simulink model "fullVehicleModel_17b"  (R2017b)
settings: Solver=VariableStepAuto  StartTime=0.0  StopTime=10.0  RelTol=1e-3
undefined symbols (not defined in the file): ambient_temp, bat, bat_r1, Batt, batt_initCharge, Batt_sensorLag_s, bvatt_AhRating, DiscIntNeverNeededParam, electronics_power, env, module_broad_area, module_small_area, module_top_area, mot, no_module, shifterPos, Ts, Ts_elec
libraries: Soft_ECUs x90, fl_lib x67, nesl_utility x29, Battery_lib x28, Gen_lib x13, simulink x10, aerolibconvert2 x7, SoftCAN_Interface x6, autolibshared x2, Additional_blocks_lib x1, elec_lib x1
(part 2 of 4)

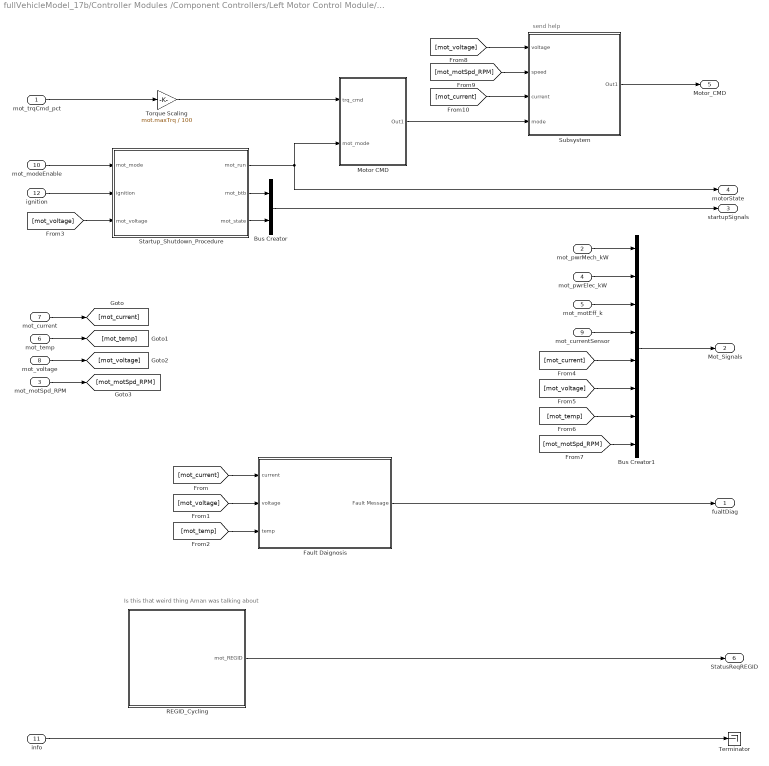
== system fullVehicleModel_17b/Controller Modules /Component Controllers/Left Motor Control Module/Controller ==
  note: send help
  note: Is this that weird thing Aman was talking about
  mot_trqCmd_pct : Inport
  mot_pwrMech_kW : Inport  Port=2
  mot_motSpd_RPM : Inport  Port=3
  mot_pwrElec_kW : Inport  Port=4
  mot_motEff_k : Inport  Port=5
  mot_temp : Inport  Port=6
  mot_current : Inport  Port=7
  mot_voltage : Inport  Port=8
  mot_currentSensor : Inport  Port=9
  mot_modeEnable : Inport  Port=10
  info : Inport  Port=11
  ignition : Inport  Port=12
  Bus Creator : BusCreator  Inputs=2
  Bus Creator1 : BusCreator  Inputs=8
  Fault Daignosis : Subsystem  AncestorBlock=Soft_ECUs/softECU_Motor/Fault Daignosis
  Motor CMD : Subsystem
  REGID_Cycling : Stateflow chart  TreatAsAtomicUnit=on
  Startup_Shutdown_Procedure : Stateflow chart  AncestorBlock=Soft_ECUs/softECU_Motor/Startup_Shutdown_Procedure  TreatAsAtomicUnit=on
  Subsystem : Subsystem
  Terminator : Terminator
  Torque Scaling : Gain  Gain=mot.maxTrq / 100
  fualtDiag : Outport
  Mot_Signals : Outport  Port=2
  startupSignals : Outport  Port=3
  motorState : Outport  Port=4
  Motor_CMD : Outport  Port=5
  StatusReqREGID : Outport  Port=6
  wires:
  mot_modeEnable/1 -> Startup_Shutdown_Procedure/1(mot_mode)
  ignition/1 -> Startup_Shutdown_Procedure/2(ignition)
  mot_trqCmd_pct/1 -> Torque Scaling/1
  Torque Scaling/1 -> Motor CMD/1(trq_cmd)
  Motor CMD/1(Out1) -> Subsystem/4(mode)
  Startup_Shutdown_Procedure/1(mot_run) -> motorState/1, Motor CMD/2(mot_mode)
  Fault Daignosis/1(Fault Message) -> fualtDiag/1
  Subsystem/1(Out1) -> Motor_CMD/1
  Startup_Shutdown_Procedure/2(mot_btb) -> Bus Creator/1
  Startup_Shutdown_Procedure/3(mot_state) -> Bus Creator/2
  Bus Creator/1 -> startupSignals/1
  REGID_Cycling/1(mot_REGID) -> StatusReqREGID/1
  mot_current/1 -> [mot_current]
  mot_voltage/1 -> [mot_voltage]
  mot_temp/1 -> [mot_temp]
  mot_motSpd_RPM/1 -> [mot_motSpd_RPM]
  mot_pwrMech_kW/1 -> Bus Creator1/1
  [mot_current] -> Fault Daignosis/1(current)
  mot_currentSensor/1 -> Bus Creator1/4
  mot_pwrElec_kW/1 -> Bus Creator1/2
  mot_motEff_k/1 -> Bus Creator1/3
  [mot_voltage] -> Fault Daignosis/2(voltage)
  [mot_temp] -> Fault Daignosis/3(temp)
  [mot_voltage] -> Startup_Shutdown_Procedure/3(mot_voltage)
  Bus Creator1/1 -> Mot_Signals/1
  [mot_current] -> Bus Creator1/5
  [mot_voltage] -> Bus Creator1/6
  [mot_temp] -> Bus Creator1/7
  [mot_motSpd_RPM] -> Bus Creator1/8
  [mot_voltage] -> Subsystem/1(voltage)
  [mot_motSpd_RPM] -> Subsystem/2(speed)
  [mot_current] -> Subsystem/3(current)
  info/1 -> Terminator/1

== system fullVehicleModel_17b/Controller Modules /Component Controllers/Left Motor Control Module/Controller Inputs ==
  note: 1) Add Subsystem or Model blocks as valid variant choices.
      | 2) You cannot connect blocks at this level. At simulation, connectivity is automatically
      | determined, based on the active variant and port name matching.
  HSC Inputs : Inport
  Motor Signals : Inport  Port=2
  Ignition : Inport  Port=3
  SiL Inputs : Subsystem  VariantControl=Variant
  mot_trqCmd_pct : Outport
  mot_pwrMech_kW : Outport  Port=2
  mot_motSpd_RPM : Outport  Port=3
  mot_pwrElec_kW : Outport  Port=4
  mot_motEff_k : Outport  Port=5
  mot_temp : Outport  Port=6
  mot_current : Outport  Port=7
  mot_voltage : Outport  Port=8
  mot_currentSensor : Outport  Port=9
  mot_modeEnable : Outport  Port=10
  Info : Outport  Port=11
  Ignition1 : Outport  Port=12

== system fullVehicleModel_17b/Controller Modules /Component Controllers/Left Motor Control Module/Controller Outputs ==
  note: 1) Add Subsystem or Model blocks as valid variant choices.
      | 2) You cannot connect blocks at this level. At simulation, connectivity is automatically
      | determined, based on the active variant and port name matching.
  FaultDiagnos : Inport
  MotorSignals : Inport  Port=2
  StartupSignals : Inport  Port=3
  MotorState : Inport  Port=4
  MotorCMD : Inport  Port=5
  StatusRequest : Inport  Port=6
  SiL Controller Outputs : Subsystem  VariantControl=Variant
  MotorToHSC : Outport
  MotorTrqCMD : Outport  Port=2

== system fullVehicleModel_17b/Controller Modules /Component Controllers/Right Motor Control Module/Controller Inputs ==
  note: 1) Add Subsystem or Model blocks as valid variant choices.
      | 2) You cannot connect blocks at this level. At simulation, connectivity is automatically
      | determined, based on the active variant and port name matching.
  In1 : Inport
  In2 : Inport  Port=2
  In3 : Inport  Port=3
  SiL Inputs : Subsystem  VariantControl=Variant
  Out1 : Outport
  Out2 : Outport  Port=2
  Out3 : Outport  Port=3
  Out4 : Outport  Port=4
  Out5 : Outport  Port=5
  Out6 : Outport  Port=6
  Out7 : Outport  Port=7
  Out8 : Outport  Port=8
  Out9 : Outport  Port=9
  Out10 : Outport  Port=10
  Out11 : Outport  Port=11
  Out12 : Outport  Port=12

== system fullVehicleModel_17b/Controller Modules /Component Controllers/Right Motor Control Module/Controller Outputs ==
  note: 1) Add Subsystem or Model blocks as valid variant choices.
      | 2) You cannot connect blocks at this level. At simulation, connectivity is automatically
      | determined, based on the active variant and port name matching.
  FaultDiagnos : Inport
  MotorSignals : Inport  Port=2
  StartupSignals : Inport  Port=3
  MotorState : Inport  Port=4
  MotorCMD : Inport  Port=5
  StatusRequest : Inport  Port=6
  SiL Controller Outputs : Subsystem  VariantControl=Variant
  MotorToHSC : Outport
  MotorTrqCMD : Outport  Port=2

== system fullVehicleModel_17b/Controller Modules /Component Controllers/Right Motor Control Module/Subsystem ==
  In1 : Inport
  In2 : Inport  Port=2
  In3 : Inport  Port=3
  In4 : Inport  Port=4
  In5 : Inport  Port=5
  In6 : Inport  Port=6
  In7 : Inport  Port=7
  In8 : Inport  Port=8
  In9 : Inport  Port=9
  In10 : Inport  Port=10
  In11 : Inport  Port=11
  In12 : Inport  Port=12
  Out1 : Outport
  Out2 : Outport  Port=2
  Out3 : Outport  Port=3
  Out4 : Outport  Port=4
  Out5 : Outport  Port=5
  Out6 : Outport  Port=6

== system fullVehicleModel_17b/Longitudinal Driver/Driver Model/Driver Model/Classic Driver ==
  CmdVel : Inport
  "Grade " : Inport  Port=2
  VelFdbk : Inport  Port=3
  Longitudinal Driver : autolibshared/Longitudinal Driver  vnom=100  Kp=15  Ki=1  Kaw=.1  Kff=.05  Kg=.01  tauerr=.03
      settings: SourceProductName=Powertrain Blockset  SourceProductBaseCode=PW
  Terminator : Terminator
  AccelCmd : Outport
  BrkCmd : Outport  Port=2
  wires:
  Longitudinal Driver/3 -> BrkCmd/1
  CmdVel/1 -> Longitudinal Driver/1
  VelFdbk/1 -> Longitudinal Driver/2
  "Grade "/1 -> Longitudinal Driver/3
  Longitudinal Driver/2 -> AccelCmd/1
  Longitudinal Driver/1 -> Terminator/1

== system fullVehicleModel_17b/Longitudinal Driver/Driver Model/Driver Model/Thermostatic Driver ==
  CmdVel : Inport
  "Grade " : Inport  Port=2
  VelFdbk : Inport  Port=3
  AccelCmd : Outport
  BrkCmd : Outport  Port=2

== system fullVehicleModel_17b/Vehicle Model/Variant Subsystem/Subsystem/Battery Dynamics ==
  Batt Signals : Inport
  Bus Selector : BusSelector  OutputSignals=Batt_SOC_pct,Batt_current_A
  Charge Curve : Lookup_n-D  NumberOfTableDimensions=1  BreakpointsForDimension1=[-5:5]  Table=tanh([-5:5])  InternalRulePriority=Speed  RndMeth=Simplest  InputSameDT=on
  Discharge Curve : Lookup_n-D  NumberOfTableDimensions=1  BreakpointsForDimension1=[-5:5]  Table=tanh([-5:5])  InternalRulePriority=Speed  RndMeth=Simplest  InputSameDT=on
  Memory2 : Memory
  Memory3 : Memory
  Simulink-PS Converter4 : nesl_utility/Simulink-PS Converter  PhysicalDomain=network_engine_domain  SubClassName=ps_input  LeftPortType=input  RightPortType=output  PseudoPeriodic=off  Frequencies=[]  NoiseDistribution=none  NoiseParameters=[]  Unit=1  AffineConversion=off  FilteringAndDerivatives=provide  SimscapeFilterOrder=1  InputFilterTimeConstant=0.001  UdotUserProvided=0
  Switch2 : Switch
  Conn1 : PMIOPort  Port=1  Side=Right
  wires:
  Charge Curve/1 -> Switch2/3
  Memory2/1 -> Charge Curve/1, Discharge Curve/1
  Memory3/1 -> Switch2/2
  Bus Selector/2 -> Memory3/1  "<Batt_current_A>"
  Bus Selector/1 -> Memory2/1  "<Batt_SOC_pct>"
  Discharge Curve/1 -> Switch2/1
  Switch2/1 -> Simulink-PS Converter4/1
  Batt Signals/1 -> Bus Selector/1
  connections:
  Conn1/RConn1 -- Simulink-PS Converter4/RConn1

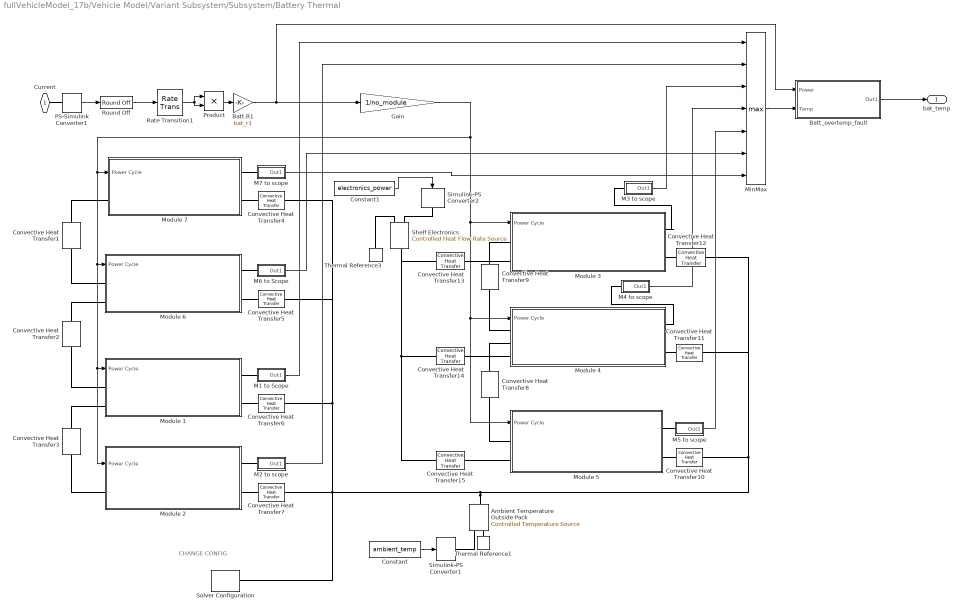
== system fullVehicleModel_17b/Vehicle Model/Variant Subsystem/Subsystem/Battery Thermal ==
  note: CHANGE CONFIG
  Ambient Temperature Outside Pack : fl_lib/Thermal/Thermal Sources/Controlled Temperature Source
      settings: SourceProductName=Simscape
  Batt.R1 : Gain  Gain=bat_r1
  Batt_overtemp_fault : Subsystem
  Constant : Constant  Value=ambient_temp
  Constant1 : Constant  Value=electronics_power
  Convective Heat Transfer1 : fl_lib/Thermal/Thermal Elements/Convective Heat Transfer  area=module_broad_area m^2  heat_tr_coeff=heat_transfer_coeff_air W/(m^2 * K)  T_specify=off  T_priority=High  T=0 K  T_nominal_specify=off  T_nominal_unit=K  T_nominal_value=1  Q_specify=off  Q_priority=High  Q=0 J/s  Q_nominal_specify=off  Q_nominal_unit=W  Q_nominal_value=1
  Convective Heat Transfer{4,7,10,12} (4 alike) : fl_lib/Thermal/Thermal Elements/Convective Heat Transfer  area=module_broad_area + 2 * (module_small_area + module_top_area) m^2  heat_tr_coeff=heat_transfer_coeff_air W/(m^2 * K)  T_specify=off  T_priority=High  T=0 K  T_nominal_specify=off  T_nominal_unit=K  T_nominal_value=1  Q_specify=off  Q_priority=High  Q=0 J/s  Q_nominal_specify=off  Q_nominal_unit=W  Q_nominal_value=1
  Convective Heat Transfer11 : fl_lib/Thermal/Thermal Elements/Convective Heat Transfer  area=2 * (module_small_area) + module_top_area m^2  heat_tr_coeff=heat_transfer_coeff_air W/(m^2 * K)  T_specify=off  T_priority=High  T=0 K  T_nominal_specify=off  T_nominal_unit=K  T_nominal_value=1  Q_specify=off  Q_priority=High  Q=0 J/s  Q_nominal_specify=off  Q_nominal_unit=W  Q_nominal_value=1
  Convective Heat Transfer{8..9,13..15} (5 alike) : fl_lib/Thermal/Thermal Elements/Convective Heat Transfer  area=module_top_area m^2  heat_tr_coeff=heat_transfer_coeff_air W/(m^2 * K)  T_specify=off  T_priority=High  T=0 K  T_nominal_specify=off  T_nominal_unit=K  T_nominal_value=1  Q_specify=off  Q_priority=High  Q=0 J/s  Q_nominal_specify=off  Q_nominal_unit=W  Q_nominal_value=1
  Convective Heat Transfer2 : fl_lib/Thermal/Thermal Elements/Convective Heat Transfer  area=module_broad_area m^2  heat_tr_coeff=heat_transfer_coeff_air W/(m^2 * K)  T_specify=off  T_priority=High  T=0 K  T_nominal_specify=off  T_nominal_unit=K  T_nominal_value=1  Q_specify=off  Q_priority=High  Q=0 J/s  Q_nominal_specify=off  Q_nominal_unit=W  Q_nominal_value=1
  Convective Heat Transfer3 : fl_lib/Thermal/Thermal Elements/Convective Heat Transfer  area=module_broad_area m^2  heat_tr_coeff=heat_transfer_coeff_air W/(m^2 * K)  T_specify=off  T_priority=High  T=0 K  T_nominal_specify=off  T_nominal_unit=K  T_nominal_value=1  Q_specify=off  Q_priority=High  Q=0 J/s  Q_nominal_specify=off  Q_nominal_unit=W  Q_nominal_value=1
  Convective Heat Transfer5 : fl_lib/Thermal/Thermal Elements/Convective Heat Transfer  area=2 * (module_small_area) + module_top_area m^2  heat_tr_coeff=heat_transfer_coeff_air W/(m^2 * K)  T_specify=off  T_priority=High  T=0 K  T_nominal_specify=off  T_nominal_unit=K  T_nominal_value=1  Q_specify=off  Q_priority=High  Q=0 J/s  Q_nominal_specify=off  Q_nominal_unit=W  Q_nominal_value=1
  Convective Heat Transfer6 : fl_lib/Thermal/Thermal Elements/Convective Heat Transfer  area=2 * (module_small_area) + module_top_area m^2  heat_tr_coeff=heat_transfer_coeff_air W/(m^2 * K)  T_specify=off  T_priority=High  T=0 K  T_nominal_specify=off  T_nominal_unit=K  T_nominal_value=1  Q_specify=off  Q_priority=High  Q=0 J/s  Q_nominal_specify=off  Q_nominal_unit=W  Q_nominal_value=1
  Gain : Gain  Gain=1/no_module
  M1 to Scope : Subsystem
  M2 to scope : Subsystem
  M3 to scope : Subsystem
  M4 to scope : Subsystem
  M5 to scope : Subsystem
  M6 to Scope : Subsystem
  M7 to scope : Subsystem
  MinMax : MinMax  Function=max  Inputs=7
  Module 1 : Subsystem
  Module 2 : Subsystem
  Module 3 : Subsystem
  Module 4 : Subsystem
  Module 5 : Subsystem
  Module 6 : Subsystem
  Module 7 : Subsystem
  PS-Simulink Converter1 : nesl_utility/PS-Simulink Converter  PhysicalDomain=network_engine_domain  SubClassName=ps_output  LeftPortType=input  RightPortType=output  PseudoPeriodic=off  Frequencies=[]  Unit=A  AffineConversion=off
  Product : Product
  Rate Transition1 : RateTransition
  Round Off : Additional_blocks_lib/Round Off
  Shelf Electronics : fl_lib/Thermal/Thermal Sources/Controlled Heat Flow Rate Source
      settings: SourceProductName=Simscape
  Simulink-PS Converter1 : nesl_utility/Simulink-PS Converter  PhysicalDomain=network_engine_domain  SubClassName=ps_input  LeftPortType=input  RightPortType=output  PseudoPeriodic=off  Frequencies=[]  NoiseDistribution=none  NoiseParameters=[]  Unit=1  AffineConversion=off  FilteringAndDerivatives=zero  SimscapeFilterOrder=1  InputFilterTimeConstant=0.001  UdotUserProvided=1
  Simulink-PS Converter2 : nesl_utility/Simulink-PS Converter  PhysicalDomain=network_engine_domain  SubClassName=ps_input  LeftPortType=input  RightPortType=output  PseudoPeriodic=off  Frequencies=[]  NoiseDistribution=none  NoiseParameters=[]  Unit=1  AffineConversion=off  FilteringAndDerivatives=zero  SimscapeFilterOrder=1  InputFilterTimeConstant=0.001  UdotUserProvided=1
  Solver Configuration : nesl_utility/Solver Configuration  PhysicalDomain=network_engine_domain  SubClassName=solver  LeftPortType=input  RightPortType=generic  Accelerate=off  Tones=[]  Harmonics=[]  SimulateNoise=off  Profile=off  UseLocalSampling=off  EnableSwitchedLinearOptims=on  FrequencyDomain=off  UseCCode=off  RelTol=0.001  AbsTol=1e-06  MinStep=1e-09  ToWorkspace=off  RevertToSquareIcSolve=off  NumHomotopyIterations=100  PhasorMode=off  PhasorModeNumHarmonics=1  DoDC=off  ResidualTolerance=1e-09  UseLocalSolver=off  LocalSolverChoice=NE_BACKWARD_EULER_ADVANCER  LocalSolverSampleTime=0.001  DoFixedCost=off  MaxNonlinIter=3  MaxModeIter=2  LinearAlgebra=Sparse  DelaysMemoryBudget=1024  AutomaticFiltering=on  FilteringTimeConstant=0.001
  Thermal Reference1 : fl_lib/Thermal/Thermal Elements/Thermal Reference
  Thermal Reference3 : fl_lib/Thermal/Thermal Elements/Thermal Reference
  Current : PMIOPort  Port=1  Side=Left
  bat_temp : Outport
  wires:
  Round Off/1 -> Rate Transition1/1
  Batt_overtemp_fault/1(Out1) -> bat_temp/1
  Gain/1 -> Module 7/1(Power Cycle), Module 6/1(Power Cycle), Module 1/1(Power Cycle), Module 2/1(Power Cycle), Module 3/1(Power Cycle), Module 4/1(Power Cycle), Module 5/1(Power Cycle)
  M2 to scope/1(Out1) -> MinMax/2
  Batt.R1/1 -> Gain/1, Batt_overtemp_fault/1(Power)
  M1 to Scope/1(Out1) -> MinMax/1
  M6 to Scope/1(Out1) -> MinMax/6
  M7 to scope/1(Out1) -> MinMax/7
  M5 to scope/1(Out1) -> MinMax/5
  M4 to scope/1(Out1) -> MinMax/4
  M3 to scope/1(Out1) -> MinMax/3
  MinMax/1 -> Batt_overtemp_fault/2(Temp)
  Constant1/1 -> Simulink-PS Converter2/1
  Constant/1 -> Simulink-PS Converter1/1
  Rate Transition1/1 -> Product/2, Product/1
  PS-Simulink Converter1/1 -> Round Off/1
  Product/1 -> Batt.R1/1
  connections:
  Module 5/RConn1 -- M5 to scope/LConn1
  Thermal Reference3/LConn1 -- Shelf Electronics/RConn2
  Convective Heat Transfer9/RConn1 -- Module 4/LConn1
  Convective Heat Transfer12/RConn1 -- Module 3/RConn2
  Module 5/LConn2 -- Convective Heat Transfer15/RConn1
  Simulink-PS Converter2/RConn1 -- Shelf Electronics/RConn1
  Convective Heat Transfer13/RConn1 -- Module 3/LConn2
  M7 to scope/LConn1 -- Module 7/RConn1
  Module 3/RConn1 -- M3 to scope/LConn1
  Module 4/LConn3 -- Convective Heat Transfer14/RConn1
  Module 4/RConn1 -- M4 to scope/LConn1
  Thermal Reference1/LConn1 -- Ambient Temperature Outside Pack/RConn2
  Convective Heat Transfer8/LConn1 -- Module 4/LConn2
  Convective Heat Transfer4/RConn1 -- Module 7/RConn2
  Convective Heat Transfer5/RConn1 -- Module 6/RConn2
  Convective Heat Transfer2/RConn1 -- Module 1/LConn1
  Module 2/RConn1 -- M2 to scope/LConn1
  Convective Heat Transfer6/RConn1 -- Module 1/RConn2
  Convective Heat Transfer3/LConn1 -- Module 1/LConn2
  Module 6/RConn1 -- M6 to Scope/LConn1
  Convective Heat Transfer11/RConn1 -- Module 4/RConn2
  Convective Heat Transfer2/LConn1 -- Module 6/LConn2
  Module 1/RConn1 -- M1 to Scope/LConn1
  Convective Heat Transfer1/RConn1 -- Module 6/LConn1
  Module 2/LConn1 -- Convective Heat Transfer3/RConn1
  Convective Heat Transfer10/RConn1 -- Module 5/RConn2
  Convective Heat Transfer8/RConn1 -- Module 5/LConn1
  Convective Heat Transfer7/RConn1 -- Module 2/RConn2
  Convective Heat Transfer1/LConn1 -- Module 7/LConn1
  Convective Heat Transfer9/LConn1 -- Module 3/LConn1
  Simulink-PS Converter1/RConn1 -- Ambient Temperature Outside Pack/RConn1
  Convective Heat Transfer14/LConn1 -- Convective Heat Transfer15/LConn1 -- Convective Heat Transfer13/LConn1 -- Shelf Electronics/LConn1
  Ambient Temperature Outside Pack/LConn1 -- Convective Heat Transfer10/LConn1 -- Convective Heat Transfer11/LConn1 -- Convective Heat Transfer12/LConn1 -- Solver Configuration/RConn1 -- Convective Heat Transfer4/LConn1 -- Convective Heat Transfer5/LConn1 -- Convective Heat Transfer6/LConn1 -- Convective Heat Transfer7/LConn1
  Current/RConn1 -- PS-Simulink Converter1/LConn1

== system fullVehicleModel_17b/Vehicle Model/Variant Subsystem/Subsystem/Input Signal Process ==
  In1 : Inport
  Contactor Cmd : Outport
  wires:
  In1/1 -> Contactor Cmd/1

== system fullVehicleModel_17b/Vehicle Model/Variant Subsystem/Subsystem/Output Signal Processing ==
  Battery Temp : Inport
  Calculations : Subsystem
  SIgnal Processing : Subsystem  Variant=on
  Voltage : PMIOPort  Port=1  Side=Left
  Current : PMIOPort  Port=2  Side=Left
  Battery Measurements : Outport
  wires:
  Calculations/4(Batt_Voltage) -> SIgnal Processing/5(Batt Voltage)
  Calculations/3(Batt_Current) -> SIgnal Processing/4(Batt Current)
  Calculations/2(Batt_SOC) -> SIgnal Processing/3(Batt SOC)
  Calculations/1(Batt_Ah) -> SIgnal Processing/2(Batt Capacity)
  Battery Temp/1 -> SIgnal Processing/1(Batt Temp)
  SIgnal Processing/1(Battery Measurements) -> Battery Measurements/1
  connections:
  Voltage/RConn1 -- Calculations/LConn1
  Current/RConn1 -- Calculations/LConn2

== system fullVehicleModel_17b/Vehicle Model/Variant Subsystem1/Subsystem/Conditional Divide ==
  u1 : Inport
  u2 : Inport  Port=2
  u3 : Inport  Port=3
  Constant1 : Constant  Value=eps
  Constant3 : Constant  Value=0
  Divide : Product  Inputs=/*
  Logical Operator : Logic  Operator=NOT  AllPortsSameDT=off  OutDataTypeStr=boolean
  Relational Operator : RelationalOperator  Operator===  OutDataTypeStr=boolean  RndMeth=Nearest
  Switch : Switch  Criteria=u2 ~= 0
  Switch1 : Switch  Criteria=u2 ~= 0
  Out1 : Outport
  wires:
  Constant3/1 -> Relational Operator/2
  Divide/1 -> Switch1/1
  u2/1 -> Relational Operator/1, Switch/3
  u1/1 -> Divide/2
  Relational Operator/1 -> Switch/2, Logical Operator/1
  u3/1 -> Switch1/3
  Constant1/1 -> Switch/1
  Switch1/1 -> Out1/1
  Logical Operator/1 -> Switch1/2
  Switch/1 -> Divide/1

== system fullVehicleModel_17b/Vehicle Model/Variant Subsystem1/Subsystem/Conditional Divide1 ==
  u1 : Inport
  u2 : Inport  Port=2
  u3 : Inport  Port=3
  Constant1 : Constant  Value=eps
  Constant3 : Constant  Value=0
  Divide : Product  Inputs=/*
  Logical Operator : Logic  Operator=NOT  AllPortsSameDT=off  OutDataTypeStr=boolean
  Relational Operator : RelationalOperator  Operator===  OutDataTypeStr=boolean  RndMeth=Nearest
  Switch : Switch  Criteria=u2 ~= 0
  Switch1 : Switch  Criteria=u2 ~= 0
  Out1 : Outport
  wires:
  Constant3/1 -> Relational Operator/2
  Divide/1 -> Switch1/1
  u2/1 -> Relational Operator/1, Switch/3
  u1/1 -> Divide/2
  Relational Operator/1 -> Switch/2, Logical Operator/1
  u3/1 -> Switch1/3
  Constant1/1 -> Switch/1
  Switch1/1 -> Out1/1
  Logical Operator/1 -> Switch1/2
  Switch/1 -> Divide/1

== system fullVehicleModel_17b/Vehicle Model/Variant Subsystem1/Subsystem/Conditional Divide2 ==
  u1 : Inport
  u2 : Inport  Port=2
  u3 : Inport  Port=3
  Constant1 : Constant  Value=eps
  Constant3 : Constant  Value=0
  Divide : Product  Inputs=/*
  Logical Operator : Logic  Operator=NOT  AllPortsSameDT=off  OutDataTypeStr=boolean
  Relational Operator : RelationalOperator  Operator===  OutDataTypeStr=boolean  RndMeth=Nearest
  Switch : Switch  Criteria=u2 ~= 0
  Switch1 : Switch  Criteria=u2 ~= 0
  Out1 : Outport
  wires:
  Constant3/1 -> Relational Operator/2
  Divide/1 -> Switch1/1
  u2/1 -> Relational Operator/1, Switch/3
  u1/1 -> Divide/2
  Relational Operator/1 -> Switch/2, Logical Operator/1
  u3/1 -> Switch1/3
  Constant1/1 -> Switch/1
  Switch1/1 -> Out1/1
  Logical Operator/1 -> Switch1/2
  Switch/1 -> Divide/1

== system fullVehicleModel_17b/Vehicle Model/Variant Subsystem1/Subsystem/Input Signal Processing ==
  note: 1) Add Subsystem or Model blocks as valid variant choices.
      | 2) You cannot connect blocks at this level. At simulation, connectivity is automatically
      | determined, based on the active variant and port name matching.
  HSC Inputs : Inport
  Genset : Inport  Port=2
  Driver : Inport  Port=3
  Subsystem : Subsystem  VariantControl=Variant
  gen_loadTrq_Nm : Outport
  gen_pwrElec_W : Outport  Port=2
  Aux Load : Outport  Port=3
  DC Mode : Outport  Port=4

== system fullVehicleModel_17b/Vehicle Model/Variant Subsystem1/Subsystem/Signal Porcessing ==
  In1 : Inport
  In2 : Inport  Port=2
  In3 : Inport  Port=3
  In4 : Inport  Port=4
  In5 : Inport  Port=5
  Bus Creator : BusCreator  Inputs=5
  Out1 : Outport
  wires:
  In4/1 -> Bus Creator/4
  Bus Creator/1 -> Out1/1
  In5/1 -> Bus Creator/5
  In2/1 -> Bus Creator/2
  In3/1 -> Bus Creator/3
  In1/1 -> Bus Creator/1

== system fullVehicleModel_17b/Vehicle Model/Variant Subsystem1/Subsystem/Signal Processing ==
  In1 : Inport
  Data Type Conversion : DataTypeConversion  OutDataTypeStr=fixdt(1,64,5)
  Data Type Conversion1 : DataTypeConversion  OutDataTypeStr=double
  Memory : Memory
  Rate Transition : RateTransition
  Out1 : Outport
  wires:
  In1/1 -> Memory/1
  Memory/1 -> Rate Transition/1
  Rate Transition/1 -> Data Type Conversion/1
  Data Type Conversion/1 -> Data Type Conversion1/1
  Data Type Conversion1/1 -> Out1/1

== system fullVehicleModel_17b/Controller Modules /Component Controllers/BMS Control Module/BMS Controller Module/BCM Constant Signals ==
  note: confusing name
  BMSAddCoolant : Constant  Value=0
  ESSCellOvervolt : Constant  Value=0  OutDataTypeStr=double
  ESSCellUndervolt : Constant  Value=0  OutDataTypeStr=double
  ESSChrgComplete : Constant  Value=0
  ESSChrgContctStatus : Constant  Value=0
  ESSLeakResistance : Constant  Value=1000
  ESSLlsStatus : Constant
  alarm : Constant  Value=0
  chargerOn : Constant  Value=0
  bcm_onPlug : Outport
  bcm_alarm : Outport  Port=2
  bcm_gfd_kOhms : Outport  Port=3
  bcm_chgDone : Outport  Port=4
  bcm_coolReq : Outport  Port=5
  bcm_chgcStat : Outport  Port=6
  bcm_llsStatus : Outport  Port=7
  bcm_cellUndervolt : Outport  Port=8
  bcm_cellOvervolt : Outport  Port=9
  wires:
  ESSChrgComplete/1 -> bcm_chgDone/1  "bcm_chgDone"
  alarm/1 -> bcm_alarm/1  "bcm_alarm"
  chargerOn/1 -> bcm_onPlug/1  "bcm_onPlug"
  ESSLeakResistance/1 -> bcm_gfd_kOhms/1  "bcm_gfd_kOhms"
  BMSAddCoolant/1 -> bcm_coolReq/1  "bcm_coolReq"
  ESSChrgContctStatus/1 -> bcm_chgcStat/1  "bcm_chgcStat"
  ESSLlsStatus/1 -> bcm_llsStatus/1  "bcm_llsStatus"
  ESSCellUndervolt/1 -> bcm_cellUndervolt/1  "bcm_cellUndervolt"
  ESSCellOvervolt/1 -> bcm_cellOvervolt/1  "bcm_cellOvervolt"

== system fullVehicleModel_17b/Controller Modules /Component Controllers/BMS Control Module/BMS Controller Module/EPO Check Enabler ==
  note: no current is passed through
  note: If charge buffer engaged
  note: Normaly battery current is passed through
  note: Or discharge buffer engaged
  Current : Inport
  charge_buf : Inport  Port=2
  discharge_buf : Inport  Port=3
  Compare To Zero : simulink/Logic and Bit Operations/Compare To Zero  relop===  OutDataTypeStr=boolean
  Compare To Zero1 : simulink/Logic and Bit Operations/Compare To Zero  relop===  OutDataTypeStr=boolean
  Constant : Constant  Value=0
  Logical Operator : Logic  Operator=OR  AllPortsSameDT=off  OutDataTypeStr=boolean
  Switch : Switch  Criteria=u2 > Threshold
  current_toEPO : Outport
  wires:
  Switch/1 -> current_toEPO/1
  charge_buf/1 -> Compare To Zero/1
  discharge_buf/1 -> Compare To Zero1/1
  Compare To Zero/1 -> Logical Operator/1
  Compare To Zero1/1 -> Logical Operator/2
  Constant/1 -> Switch/3
  Current/1 -> Switch/1
  Logical Operator/1 -> Switch/2

== system fullVehicleModel_17b/Controller Modules /Component Controllers/BMS Control Module/BMS Controller Module/EPO_Check ==
  Current : Inport
  Chg_max_amps : Inport  Port=2
  DisChg_max_amps : Inport  Port=3
  bat_temp : Inport  Port=4
  Abs1 : Abs
  Abs2 : Abs
  "Allowance " : Constant  Value=bat.currentallowance
  EPO_charge : Subsystem
  EPO_discharge : Subsystem
  Logical Operator : Logic  Operator=OR  Inputs=3  AllPortsSameDT=off  OutDataTypeStr=boolean
  Relational Operator1 : RelationalOperator  Operator=>  OutDataTypeStr=boolean  RndMeth=Nearest
  Saturation : Saturate  UpperLimit=inf  LowerLimit=0
  Saturation1 : Saturate  UpperLimit=0  LowerLimit=-inf
  Sum : Sum  Inputs=|++
  Sum1 : Sum  Inputs=|++
  Temp_Max : Constant  Value=bat.maxtemp
  EPO_BCM : Outport
  wires:
  Abs2/1 -> EPO_discharge/1(Current)
  Saturation1/1 -> Abs2/1
  Saturation/1 -> EPO_charge/1(Current)
  Logical Operator/1 -> EPO_BCM/1
  EPO_charge/1(EPO) -> Logical Operator/1
  EPO_discharge/1(EPO) -> Logical Operator/2
  Relational Operator1/1 -> Logical Operator/3
  Chg_max_amps/1 -> Sum/1, EPO_charge/2(Chg_max_amps)
  DisChg_max_amps/1 -> Abs1/1
  bat_temp/1 -> Relational Operator1/1
  Current/1 -> Saturation/1, Saturation1/1
  Temp_Max/1 -> Relational Operator1/2
  Abs1/1 -> Sum1/2, EPO_discharge/3(DIsChg_max_amps)
  "Allowance "/1 -> Sum1/1, Sum/2
  Sum/1 -> EPO_charge/3(Chg_max_plus_allowance)
  Sum1/1 -> EPO_discharge/2(max_discharge_plus_allowance)

== system fullVehicleModel_17b/Controller Modules /Component Controllers/BMS Control Module/BMS Controller Module/Subsystem ==
  note: what the hell is going on
  Current : Inport
  SOC : Inport  Port=2
  Temperature : Inport  Port=3
  Charge_Discharge_limit_maps : Subsystem
  Chg_Buffer_Calculation : Battery_lib/Buffer_Calculation
  Dis_Buffer_Calculation : Battery_lib/Buffer_Calculation
  Gain{,1..2,4} (4 alike) : Gain  Gain=-1
  Chg_Buf_pct : Outport
  DisChg_Buf_pct : Outport  Port=2
  Chg_max_A : Outport  Port=3
  DisChg_max_A : Outport  Port=4
  wires:
  Chg_Buffer_Calculation/2 -> Chg_max_A/1
  Chg_Buffer_Calculation/1 -> Chg_Buf_pct/1
  SOC/1 -> Charge_Discharge_limit_maps/2(soc %)
  Gain1/1 -> Dis_Buffer_Calculation/2
  Dis_Buffer_Calculation/1 -> DisChg_Buf_pct/1
  Dis_Buffer_Calculation/2 -> Gain4/1
  Gain2/1 -> Dis_Buffer_Calculation/3
  Charge_Discharge_limit_maps/4(dclimit) -> Gain2/1
  Charge_Discharge_limit_maps/3(dplimit) -> Gain1/1
  Charge_Discharge_limit_maps/2(cclimit) -> Chg_Buffer_Calculation/3
  Gain/1 -> Dis_Buffer_Calculation/1
  Gain4/1 -> DisChg_max_A/1
  Charge_Discharge_limit_maps/1(cplimit) -> Chg_Buffer_Calculation/2
  Temperature/1 -> Charge_Discharge_limit_maps/1(bat_temp)
  Current/1 -> Chg_Buffer_Calculation/1, Gain/1

== system fullVehicleModel_17b/Controller Modules /Component Controllers/BMS Control Module/BMS Controller Module/Subsystem1 ==
  IgnitiionCMD : Inport
  Constant : Constant
  Constant1 : Constant  Value=0
  Switch : Switch  Criteria=u2 > Threshold
  Ignition : Outport
  ignition_status : Outport  Port=2
  wires:
  Constant/1 -> Switch/1
  Constant1/1 -> Switch/3
  IgnitiionCMD/1 -> Switch/2, Ignition/1
  Switch/1 -> ignition_status/1

== system fullVehicleModel_17b/Controller Modules /Component Controllers/BMS Control Module/BMS Controller Module/contactor logic ==
  note: Not sure about the details of this logic
  hsc_epo : Inport
  contactor rqst : Inport  Port=2
  contactor_pwr_cmd : Inport  Port=3
  bcm_epo : Inport  Port=4
  Bus Creator1 : BusCreator  Inputs=3
  Contactor_actuation : Stateflow chart  TreatAsAtomicUnit=on
  EPO_Check : Stateflow chart  TreatAsAtomicUnit=on
  Logical Operator : Logic  AllPortsSameDT=off  OutDataTypeStr=boolean
  Logical Operator1 : Logic  Operator=OR  AllPortsSameDT=off  OutDataTypeStr=boolean
  contactor _signals : Outport
  contactor _status : Outport  Port=2
  wires:
  Logical Operator1/1 -> EPO_Check/1(EPO)
  bcm_epo/1 -> Logical Operator1/2
  hsc_epo/1 -> Logical Operator1/1
  Contactor_actuation/3(Pre_charge_actu) -> Bus Creator1/3  "Pre-charge_Actu"
  Bus Creator1/1 -> contactor _signals/1
  Contactor_actuation/2(Positive_actu) -> Bus Creator1/2  "Positive_Actu"
  Contactor_actuation/1(Negative_actu) -> Bus Creator1/1  "Negative_Actu"
  contactor rqst/1 -> EPO_Check/2(contactor_rqst)
  Logical Operator/1 -> contactor _status/1, Contactor_actuation/1(close_contact)
  contactor_pwr_cmd/1 -> Logical Operator/1
  EPO_Check/1(contactors) -> Logical Operator/2

== system fullVehicleModel_17b/Controller Modules /Component Controllers/BMS Control Module/Controller Inputs/SiL Inputs ==
  note: state processing
  note: Data Type
      | Conversion
  note: After this signal data
      | type should match what
      | the control code expects
  note: Many signals need
      | to be offset to correspond
      | to model values
  note: Model Units
  note: Hooray! Ready for
      | the model!
  note: Gain
  note: Offset/Bias
  note: Many signals need
      | to be scaled from
      | hardware values
  note: These subsystems can be used
      |  to override the received HW value
      | of a signal to a constant value
  note: Raw Signals
      | From Hardware
  note: Override Switch
  BattHSC : Inport
  BattPlant : Inport  Port=2
  IgnitionCMD : Inport  Port=3
  Bus Selector1 : BusSelector  OutputSignals=Current,SOC,Batt_Temp_C,Voltage
  Bus Selector3 : BusSelector  OutputSignals=hsc_bcmEnable,hsc_bcm_epo,hsc_maincClose
  Conversion_setBmsEnable : DataTypeConversion  OutDataTypeStr=boolean
  Conversion_setBmsEpo : DataTypeConversion  OutDataTypeStr=boolean
  Conversion_setBmsMainContactorClose : DataTypeConversion  OutDataTypeStr=boolean
  Override_setBmsEnable : Battery_lib/BMS/SoftECU_BMS_Rx_SetterConversion1/Override_setBmsEnable
  Override_setBmsEpo : Battery_lib/BMS/SoftECU_BMS_Rx_SetterConversion1/Override_setBmsEpo
  Override_setBmsMainContactorClose : Battery_lib/BMS/SoftECU_BMS_Rx_SetterConversion1/Override_setBmsMainContactorClose
  Rate Transition : RateTransition
  BMS_BMSEnable : Outport
  BMS_BMSEPO : Outport  Port=2
  BMS_mainContctClose : Outport  Port=3
  Batt_current_A : Outport  Port=4
  Batt_SOC_pct : Outport  Port=5
  Batt_temp_C : Outport  Port=6
  Batt_voltage_V : Outport  Port=7
  IngnitionCMD : Outport  Port=8
  wires:
  Override_setBmsMainContactorClose/1 -> BMS_mainContctClose/1  "setBmsMainContactorClose[bool]"
  BattHSC/1 -> Bus Selector3/1
  Conversion_setBmsEnable/1 -> Override_setBmsEnable/1
  Override_setBmsEnable/1 -> BMS_BMSEnable/1  "setBmsEnable[bool]"
  Conversion_setBmsEpo/1 -> Override_setBmsEpo/1
  Conversion_setBmsMainContactorClose/1 -> Override_setBmsMainContactorClose/1
  Bus Selector3/2 -> Conversion_setBmsEpo/1  "<hsc_bcm_epo>"
  Bus Selector3/1 -> Conversion_setBmsEnable/1  "<hsc_bcmEnable>"
  Override_setBmsEpo/1 -> BMS_BMSEPO/1  "setBmsEpo[bool]"
  Bus Selector3/3 -> Conversion_setBmsMainContactorClose/1  "<hsc_maincClose>"
  BattPlant/1 -> Rate Transition/1
  Bus Selector1/3 -> Batt_temp_C/1  "<Batt_Temp_C>"
  Bus Selector1/1 -> Batt_current_A/1  "<Current>"
  Rate Transition/1 -> Bus Selector1/1
  Bus Selector1/2 -> Batt_SOC_pct/1  "<SOC>"
  Bus Selector1/4 -> Batt_voltage_V/1  "<Voltage>"
  IgnitionCMD/1 -> IngnitionCMD/1

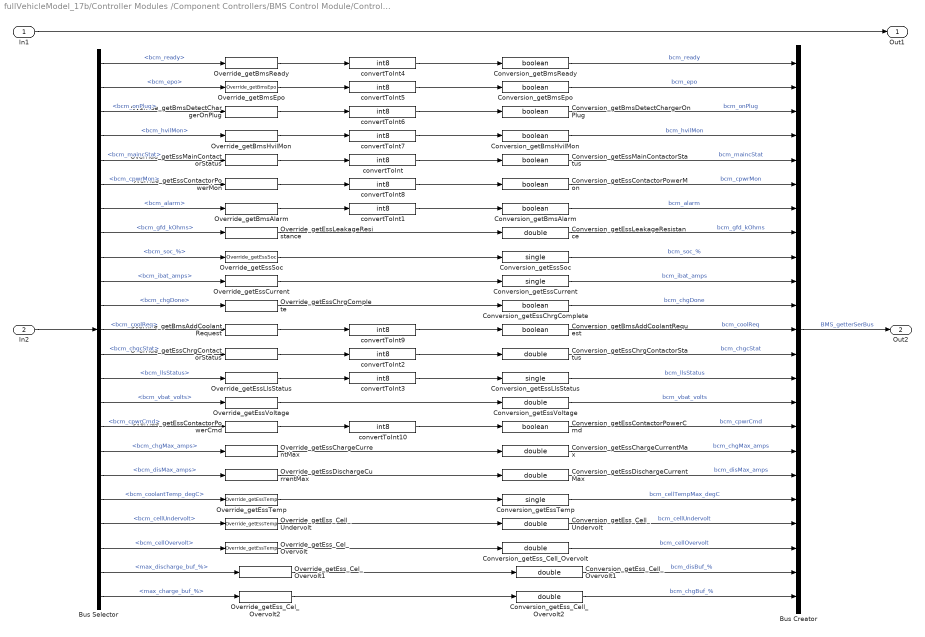
== system fullVehicleModel_17b/Controller Modules /Component Controllers/BMS Control Module/Controller Outputs/SiL Controller Outputs ==
  In1 : Inport
  In2 : Inport  Port=2
  Bus Creator : BusCreator  Inputs=23
  Bus Selector : BusSelector  OutputSignals=bcm_ready,bcm_epo,bcm_onPlug,bcm_hvilMon,bcm_maincStat,bcm_cpwrMon,bcm_alarm,bcm_gfd_kOhms,bcm_soc_%,bcm_ibat_amps,bcm_chgDone,bcm_coolReq,bcm_chgcStat,bcm_llsStatus,bcm_vbat_volts,bcm_cpwrCmd,bcm_chgMax_amps,bcm_disMax_amps,bcm_coolantTemp_degC,bcm_cellUndervolt,bcm_cellOvervolt,max_discharge_buf_%,max_charge_buf_%
  Conversion_getBmsAddCoolantRequest : DataTypeConversion  OutDataTypeStr=boolean
  Conversion_getBmsAlarm : DataTypeConversion  OutDataTypeStr=boolean
  Conversion_getBmsDetectChargerOnPlug : DataTypeConversion  OutDataTypeStr=boolean
  Conversion_getBmsEpo : DataTypeConversion  OutDataTypeStr=boolean
  Conversion_getBmsHvilMon : DataTypeConversion  OutDataTypeStr=boolean
  Conversion_getBmsReady : DataTypeConversion  OutDataTypeStr=boolean
  Conversion_getEssChargeCurrentMax : DataTypeConversion  OutDataTypeStr=double
  Conversion_getEssChrgComplete : DataTypeConversion  OutDataTypeStr=boolean
  Conversion_getEssChrgContactorStatus : DataTypeConversion  OutDataTypeStr=double
  Conversion_getEssContactorPowerCmd : DataTypeConversion  OutDataTypeStr=boolean
  Conversion_getEssContactorPowerMon : DataTypeConversion  OutDataTypeStr=boolean
  Conversion_getEssCurrent : DataTypeConversion  OutDataTypeStr=single
  Conversion_getEssDischargeCurrentMax : DataTypeConversion  OutDataTypeStr=double
  Conversion_getEssLeakageResistance : DataTypeConversion  OutDataTypeStr=double
  Conversion_getEssLlsStatus : DataTypeConversion  OutDataTypeStr=single
  Conversion_getEssMainContactorStatus : DataTypeConversion  OutDataTypeStr=boolean
  Conversion_getEssSoc : DataTypeConversion  OutDataTypeStr=single
  Conversion_getEssTemp : DataTypeConversion  OutDataTypeStr=single
  Conversion_getEssVoltage : DataTypeConversion  OutDataTypeStr=double
  Conversion_getEss_Cell_Overvolt : DataTypeConversion  OutDataTypeStr=double
  Conversion_getEss_Cell_Overvolt1 : DataTypeConversion  OutDataTypeStr=double
  Conversion_getEss_Cell_Overvolt2 : DataTypeConversion  OutDataTypeStr=double
  Conversion_getEss_Cell_Undervolt : DataTypeConversion  OutDataTypeStr=double
  Override_getBmsAddCoolantRequest : Battery_lib/BMS/SoftECU_BMS_Tx_GetterConversion/Override_getBmsAddCoolantRequest
  Override_getBmsAlarm : Battery_lib/BMS/SoftECU_BMS_Tx_GetterConversion/Override_getBmsAlarm
  Override_getBmsDetectChargerOnPlug : Battery_lib/BMS/SoftECU_BMS_Tx_GetterConversion/Override_getBmsDetectChargerOnPlug
  Override_getBmsEpo : Battery_lib/BMS/SoftECU_BMS_Tx_GetterConversion/Override_getBmsEpo
  Override_getBmsHvilMon : Battery_lib/BMS/SoftECU_BMS_Tx_GetterConversion/Override_getBmsHvilMon
  Override_getBmsReady : Battery_lib/BMS/SoftECU_BMS_Tx_GetterConversion/Override_getBmsReady
  Override_getEssChargeCurrentMax : Battery_lib/BMS/SoftECU_BMS_Tx_GetterConversion/Override_getEssChargeCurrentMax
  Override_getEssChrgComplete : Battery_lib/BMS/SoftECU_BMS_Tx_GetterConversion/Override_getEssChrgComplete
  Override_getEssChrgContactorStatus : Battery_lib/BMS/SoftECU_BMS_Tx_GetterConversion/Override_getEssChrgContactorStatus
  Override_getEssContactorPowerCmd : Battery_lib/BMS/SoftECU_BMS_Tx_GetterConversion/Override_getEssContactorPowerCmd
  Override_getEssContactorPowerMon : Battery_lib/BMS/SoftECU_BMS_Tx_GetterConversion/Override_getEssContactorPowerMon
  Override_getEssCurrent : Battery_lib/BMS/SoftECU_BMS_Tx_GetterConversion/Override_getEssCurrent
  Override_getEssDischargeCurrentMax : Battery_lib/BMS/SoftECU_BMS_Tx_GetterConversion/Override_getEssDischargeCurrentMax
  Override_getEssLeakageResistance : Battery_lib/BMS/SoftECU_BMS_Tx_GetterConversion/Override_getEssLeakageResistance
  Override_getEssLlsStatus : Battery_lib/BMS/SoftECU_BMS_Tx_GetterConversion/Override_getEssLlsStatus
  Override_getEssMainContactorStatus : Battery_lib/BMS/SoftECU_BMS_Tx_GetterConversion/Override_getEssMainContactorStatus
  Override_getEssSoc : Battery_lib/BMS/SoftECU_BMS_Tx_GetterConversion/Override_getEssSoc
  Override_getEssTemp : Battery_lib/BMS/SoftECU_BMS_Tx_GetterConversion/Override_getEssTemp
  Override_getEssVoltage : Battery_lib/BMS/SoftECU_BMS_Tx_GetterConversion/Override_getEssVoltage
  Override_getEss_Cel_Overvolt : Battery_lib/BMS/SoftECU_BMS_Tx_GetterConversion/Override_getEssTemp
  Override_getEss_Cel_Overvolt1 : Battery_lib/BMS/SoftECU_BMS_Tx_GetterConversion/Override_getEss_Cel_Overvolt1
  Override_getEss_Cel_Overvolt2 : Battery_lib/BMS/SoftECU_BMS_Tx_GetterConversion/Override_getEss_Cel_Overvolt2
  Override_getEss_Cell_Undervolt : Battery_lib/BMS/SoftECU_BMS_Tx_GetterConversion/Override_getEssTemp
  convertToInt{,1..10} (11 alike) : DataTypeConversion  OutDataTypeStr=int8
  Out1 : Outport
  Out2 : Outport  Port=2
  wires:
  Bus Selector/21 -> Override_getEss_Cel_Overvolt/1  "<bcm_cellOvervolt>"
  Bus Selector/2 -> Override_getBmsEpo/1  "<bcm_epo>"
  Conversion_getBmsAlarm/1 -> Bus Creator/7  "bcm_alarm"
  Bus Selector/3 -> Override_getBmsDetectChargerOnPlug/1  "<bcm_onPlug>"
  Conversion_getEssContactorPowerMon/1 -> Bus Creator/6  "bcm_cpwrMon"
  Conversion_getEss_Cell_Overvolt2/1 -> Bus Creator/23  "bcm_chgBuf_%"
  Conversion_getBmsHvilMon/1 -> Bus Creator/4  "bcm_hvilMon"
  Conversion_getBmsDetectChargerOnPlug/1 -> Bus Creator/3  "bcm_onPlug"
  convertToInt9/1 -> Conversion_getBmsAddCoolantRequest/1
  Conversion_getBmsEpo/1 -> Bus Creator/2  "bcm_epo"
  Bus Selector/5 -> Override_getEssMainContactorStatus/1  "<bcm_maincStat>"
  Conversion_getEssChrgContactorStatus/1 -> Bus Creator/13  "bcm_chgcStat"
  Conversion_getBmsAddCoolantRequest/1 -> Bus Creator/12  "bcm_coolReq"
  Conversion_getEssChrgComplete/1 -> Bus Creator/11  "bcm_chgDone"
  Conversion_getEssCurrent/1 -> Bus Creator/10  "bcm_ibat_amps"
  Conversion_getEss_Cell_Overvolt/1 -> Bus Creator/21  "bcm_cellOvervolt"
  convertToInt5/1 -> Conversion_getBmsEpo/1
  convertToInt6/1 -> Conversion_getBmsDetectChargerOnPlug/1
  convertToInt8/1 -> Conversion_getEssContactorPowerMon/1
  Override_getBmsDetectChargerOnPlug/1 -> convertToInt6/1
  convertToInt2/1 -> Conversion_getEssChrgContactorStatus/1
  Bus Selector/11 -> Override_getEssChrgComplete/1  "<bcm_chgDone>"
  convertToInt/1 -> Conversion_getEssMainContactorStatus/1
  convertToInt1/1 -> Conversion_getBmsAlarm/1
  Bus Selector/23 -> Override_getEss_Cel_Overvolt2/1  "<max_charge_buf_%>"
  Conversion_getEss_Cell_Overvolt1/1 -> Bus Creator/22  "bcm_disBuf_%"
  Override_getBmsAlarm/1 -> convertToInt1/1
  Override_getEss_Cel_Overvolt1/1 -> Conversion_getEss_Cell_Overvolt1/1
  Bus Selector/15 -> Override_getEssVoltage/1  "<bcm_vbat_volts>"
  Bus Selector/12 -> Override_getBmsAddCoolantRequest/1  "<bcm_coolReq>"
  Override_getEssContactorPowerCmd/1 -> convertToInt10/1
  Override_getBmsEpo/1 -> convertToInt5/1
  Bus Selector/14 -> Override_getEssLlsStatus/1  "<bcm_llsStatus>"
  convertToInt10/1 -> Conversion_getEssContactorPowerCmd/1
  Bus Selector/9 -> Override_getEssSoc/1  "<bcm_soc_%>"
  Override_getEss_Cell_Undervolt/1 -> Conversion_getEss_Cell_Undervolt/1
  Bus Selector/7 -> Override_getBmsAlarm/1  "<bcm_alarm>"
  Override_getEssMainContactorStatus/1 -> convertToInt/1
  Bus Selector/8 -> Override_getEssLeakageResistance/1  "<bcm_gfd_kOhms>"
  Override_getEss_Cel_Overvolt/1 -> Conversion_getEss_Cell_Overvolt/1
  Conversion_getEssContactorPowerCmd/1 -> Bus Creator/16  "bcm_cpwrCmd"
  Conversion_getEssSoc/1 -> Bus Creator/9  "bcm_soc_%"
  Bus Selector/6 -> Override_getEssContactorPowerMon/1  "<bcm_cpwrMon>"
  Override_getEssLeakageResistance/1 -> Conversion_getEssLeakageResistance/1
  Override_getEssCurrent/1 -> Conversion_getEssCurrent/1
  Override_getEssSoc/1 -> Conversion_getEssSoc/1
  Override_getEssContactorPowerMon/1 -> convertToInt8/1
  Override_getBmsHvilMon/1 -> convertToInt7/1
  Conversion_getEssMainContactorStatus/1 -> Bus Creator/5  "bcm_maincStat"
  Override_getEss_Cel_Overvolt2/1 -> Conversion_getEss_Cell_Overvolt2/1
  In2/1 -> Bus Selector/1
  Conversion_getEssTemp/1 -> Bus Creator/19  "bcm_cellTempMax_degC"
  Conversion_getBmsReady/1 -> Bus Creator/1  "bcm_ready"
  Override_getEssChrgContactorStatus/1 -> convertToInt2/1
  Bus Selector/19 -> Override_getEssTemp/1  "<bcm_coolantTemp_degC>"
  Bus Selector/17 -> Override_getEssChargeCurrentMax/1  "<bcm_chgMax_amps>"
  Override_getEssChrgComplete/1 -> Conversion_getEssChrgComplete/1
  Bus Selector/1 -> Override_getBmsReady/1  "<bcm_ready>"
  Conversion_getEssVoltage/1 -> Bus Creator/15  "bcm_vbat_volts"
  Override_getEssVoltage/1 -> Conversion_getEssVoltage/1
  Bus Selector/4 -> Override_getBmsHvilMon/1  "<bcm_hvilMon>"
  Override_getEssTemp/1 -> Conversion_getEssTemp/1
  Override_getBmsAddCoolantRequest/1 -> convertToInt9/1
  Override_getEssChargeCurrentMax/1 -> Conversion_getEssChargeCurrentMax/1
  Override_getBmsReady/1 -> convertToInt4/1
  Bus Selector/18 -> Override_getEssDischargeCurrentMax/1  "<bcm_disMax_amps>"
  Conversion_getEss_Cell_Undervolt/1 -> Bus Creator/20  "bcm_cellUndervolt"
  Conversion_getEssDischargeCurrentMax/1 -> Bus Creator/18  "bcm_disMax_amps"
  Bus Selector/13 -> Override_getEssChrgContactorStatus/1  "<bcm_chgcStat>"
  convertToInt7/1 -> Conversion_getBmsHvilMon/1
  Bus Selector/10 -> Override_getEssCurrent/1  "<bcm_ibat_amps>"
  Bus Selector/16 -> Override_getEssContactorPowerCmd/1  "<bcm_cpwrCmd>"
  convertToInt4/1 -> Conversion_getBmsReady/1
  convertToInt3/1 -> Conversion_getEssLlsStatus/1
  Bus Selector/22 -> Override_getEss_Cel_Overvolt1/1  "<max_discharge_buf_%>"
  Override_getEssDischargeCurrentMax/1 -> Conversion_getEssDischargeCurrentMax/1
  Bus Selector/20 -> Override_getEss_Cell_Undervolt/1  "<bcm_cellUndervolt>"
  Conversion_getEssLlsStatus/1 -> Bus Creator/14  "bcm_llsStatus"
  Conversion_getEssLeakageResistance/1 -> Bus Creator/8  "bcm_gfd_kOhms"
  Bus Creator/1 -> Out2/1  "BMS_getterSerBus"
  Override_getEssLlsStatus/1 -> convertToInt3/1
  Conversion_getEssChargeCurrentMax/1 -> Bus Creator/17  "bcm_chgMax_amps"
  In1/1 -> Out1/1

== system fullVehicleModel_17b/Controller Modules /Component Controllers/Genset Control Module/Controller Inputs/HiL Inputs ==
  HSCCmd : Inport
  VehPlant : Inport  Port=2
  Bus Selector : BusSelector  OutputSignals=eng_starterSwitchReq_bool,eng_killSwitchReq_bool,eng_powerSupplyReq_bool,eng_status_val,eng_throttleReq_pct,gen_enable
  Bus Selector1 : BusSelector  OutputSignals=P_elec_kW,eng_engineSpd_RPM,eng_totFuelConsumption_L
  Bus Selector2 : BusSelector  OutputSignals=eng_comp_sig,gen_comp_sig
  Bus Selector3 : BusSelector  OutputSignals=gen_loadTrqReq_Nm
  Compare To Constant : simulink/Logic and Bit Operations/Compare To Constant  relop=<=  const=6.75  OutDataTypeStr=boolean
  Gain : Gain  Gain=0.264712
  eng_starterSwitchReq_bool : Outport
  Out2 : Outport  Port=2
  Out3 : Outport  Port=3
  Out4 : Outport  Port=4
  Out5 : Outport  Port=5
  Out6 : Outport  Port=6
  Out7 : Outport  Port=7
  Out8 : Outport  Port=8
  Out9 : Outport  Port=9
  Out10 : Outport  Port=10
  wires:
  VehPlant/1 -> Bus Selector1/1
  Bus Selector/4 -> Out4/1  "<eng_status_val>"
  Bus Selector/3 -> Out3/1  "<eng_powerSupplyReq_bool>"
  Compare To Constant/1 -> Out10/1  "eng_fuelLevelBit_bool"
  HSCCmd/1 -> Bus Selector2/1
  Bus Selector2/2 -> Bus Selector3/1  "<gen_comp_sig>"
  Bus Selector2/1 -> Bus Selector/1  "<eng_comp_sig>"
  Bus Selector1/1 -> Out8/1  "<P_elec_kW>"
  Bus Selector1/3 -> Gain/1  "<eng_totFuelConsumption_L>"
  Bus Selector1/2 -> Out9/1  "<eng_engineSpd_RPM>"
  Bus Selector3/1 -> Out7/1  "<gen_loadTrqReq_Nm>"
  Bus Selector/5 -> Out5/1  "<eng_throttleReq_pct>"
  Bus Selector/6 -> Out6/1  "<gen_enable>"
  Gain/1 -> Compare To Constant/1  "US_Gallons"
  Bus Selector/1 -> eng_starterSwitchReq_bool/1  "<eng_starterSwitchReq_bool>"
  Bus Selector/2 -> Out2/1  "<eng_killSwitchReq_bool>"

== system fullVehicleModel_17b/Controller Modules /Component Controllers/Genset Control Module/Controller Inputs/SiL Inputs ==
  HSCCmd : Inport
  VehPlant : Inport  Port=2
  Bus Selector : BusSelector  OutputSignals=eng_starterSwitchReq_bool,eng_killSwitchReq_bool,eng_powerSupplyReq_bool,eng_status_val,eng_throttleReq_pct,gen_enable
  Bus Selector1 : BusSelector  OutputSignals=P_elec_kW,eng_engineSpd_RPM,eng_totFuelConsumption_L
  Bus Selector2 : BusSelector  OutputSignals=eng_comp_sig,gen_comp_sig
  Bus Selector3 : BusSelector  OutputSignals=gen_loadTrqReq_Nm
  Compare To Constant : simulink/Logic and Bit Operations/Compare To Constant  relop=<=  const=6.75  OutDataTypeStr=boolean
  Gain : Gain  Gain=0.264712
  eng_starterSwitchReq_bool : Outport
  Out2 : Outport  Port=2
  Out3 : Outport  Port=3
  Out4 : Outport  Port=4
  Out5 : Outport  Port=5
  Out6 : Outport  Port=6
  Out7 : Outport  Port=7
  Out8 : Outport  Port=8
  Out9 : Outport  Port=9
  Out10 : Outport  Port=10
  wires:
  Bus Selector/5 -> Out5/1  "<eng_throttleReq_pct>"
  Bus Selector/2 -> Out2/1  "<eng_killSwitchReq_bool>"
  Bus Selector/3 -> Out3/1  "<eng_powerSupplyReq_bool>"
  Bus Selector/6 -> Out6/1  "<gen_enable>"
  Bus Selector2/2 -> Bus Selector3/1  "<gen_comp_sig>"
  HSCCmd/1 -> Bus Selector2/1
  Bus Selector2/1 -> Bus Selector/1  "<eng_comp_sig>"
  Bus Selector/1 -> eng_starterSwitchReq_bool/1  "<eng_starterSwitchReq_bool>"
  Bus Selector/4 -> Out4/1  "<eng_status_val>"
  Bus Selector3/1 -> Out7/1  "<gen_loadTrqReq_Nm>"
  Bus Selector1/3 -> Gain/1  "<eng_totFuelConsumption_L>"
  VehPlant/1 -> Bus Selector1/1
  Bus Selector1/1 -> Out8/1  "<P_elec_kW>"
  Compare To Constant/1 -> Out10/1  "eng_fuelLevelBit_bool"
  Gain/1 -> Compare To Constant/1  "US_Gallons"
  Bus Selector1/2 -> Out9/1  "<eng_engineSpd_RPM>"

== system fullVehicleModel_17b/Controller Modules /Component Controllers/Genset Control Module/Controller Outputs/SiL Controller Outputs ==
  eng_enable : Inport
  eng_throttleReq_pct : Inport  Port=2
  gen_enable : Inport  Port=3
  gen_loadTrqReq_Nm : Inport  Port=4
  gen_pwrElec_kW : Inport  Port=5
  eng_engineSpd_rpm : Inport  Port=6
  eng_fuelLevelBit_bool : Inport  Port=7
  Bus Creator : BusCreator  Inputs=4
  Bus Creator1 : BusCreator  Inputs=3
  PlantCmds : Outport
  ToHSC : Outport  Port=2
  wires:
  eng_enable/1 -> Bus Creator/1  "enableSig"
  gen_loadTrqReq_Nm/1 -> Bus Creator/4
  eng_throttleReq_pct/1 -> Bus Creator/2
  Bus Creator/1 -> PlantCmds/1
  gen_enable/1 -> Bus Creator/3
  Bus Creator1/1 -> ToHSC/1  "genset_SoftECU"
  eng_engineSpd_rpm/1 -> Bus Creator1/2
  gen_pwrElec_kW/1 -> Bus Creator1/1
  eng_fuelLevelBit_bool/1 -> Bus Creator1/3  "eng_fuelLevelBit_bool"

== system fullVehicleModel_17b/Controller Modules /Component Controllers/Genset Control Module/Genset Controller Module/Engine Enable System ==
  In1 : Inport
  In2 : Inport  Port=2
  In3 : Inport  Port=3
  In4 : Inport  Port=4
  Out1 : Outport
